simulink model "q4_week1"  (R2024b)
settings: Solver=VariableStepAuto  StartTime=0.0  StopTime=10.0  RelTol=1e-3
settings Model: Creator=Sagar  LastModifiedBy=Sagar

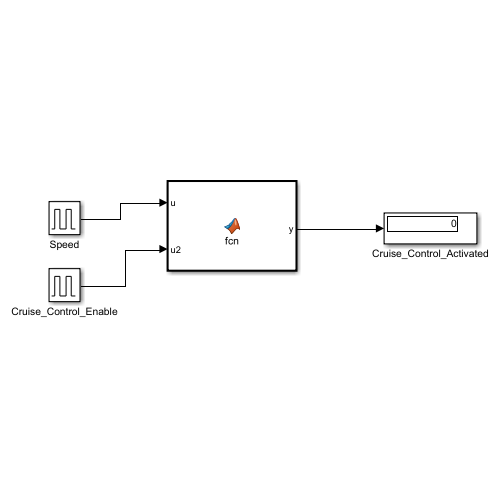
[thumbnail: Simulink's stored preview of the top-level diagram]
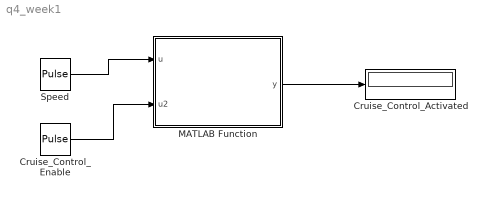
== system q4_week1 ==
  Cruise_Control_Activated : Display
  Cruise_Control_Enable : DiscretePulseGenerator  PulseType=Time based  Period=3  PulseWidth=10
  MATLAB Function : MATLAB Function  TreatAsAtomicUnit=on
  Speed : DiscretePulseGenerator  PulseType=Time based  Amplitude=65  PulseWidth=50
  wires:
  Speed/1 -> MATLAB Function/1(u)
  Cruise_Control_Enable/1 -> MATLAB Function/2(u2)
  MATLAB Function/1(y) -> Cruise_Control_Activated/1

== matlab function q4_week1/MATLAB Function ==
  data: u input; y output; u2 input
function y = fcn(u, u2)
%#codegen
if u2>0 & u >60
    y=1
else
    y=0
end
